simulink model "bicycle"  (R2025b)
settings: Solver=VariableStepAuto  StartTime=0.0  StopTime=10.0  RelTol=1e-3
undefined symbols (not defined in the file): vehicle
settings Model: Creator=jaiden  LastModifiedBy=jaiden

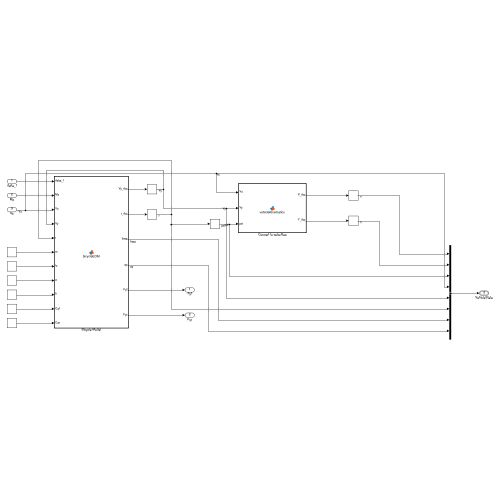
[thumbnail: Simulink's stored preview of the top-level diagram]
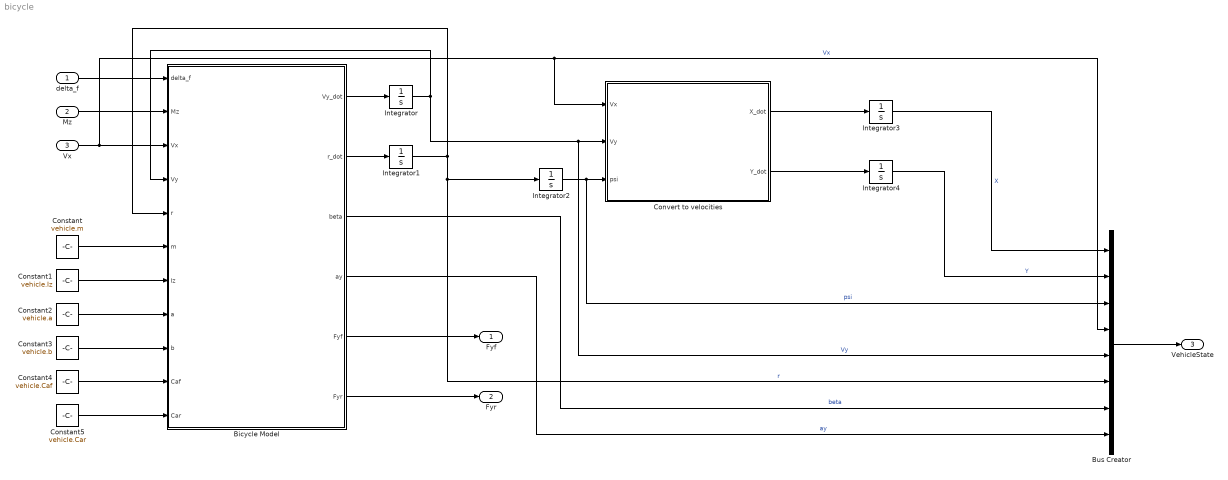
== system bicycle ==
  delta_f : Inport
  Mz : Inport  Port=2
  Vx : Inport  Port=3
  Bicycle Model : MATLAB Function  TreatAsAtomicUnit=on
  Bus Creator : BusCreator  Inputs=8  OutDataTypeStr=Bus: VehicleStateBus
  Constant : Constant  Value=vehicle.m  VectorParams1D=off
  Constant1 : Constant  Value=vehicle.Iz
  Constant2 : Constant  Value=vehicle.a
  Constant3 : Constant  Value=vehicle.b
  Constant4 : Constant  Value=vehicle.Caf
  Constant5 : Constant  Value=vehicle.Car
  Convert to velocities : MATLAB Function  TreatAsAtomicUnit=on
  Integrator{,1..4} (5 alike) : Integrator
  Fyf : Outport
  Fyr : Outport  Port=2
  VehicleState : Outport  Port=3  OutDataTypeStr=Bus: VehicleStateBus
  wires:
  delta_f/1 -> Bicycle Model/1(delta_f)
  Mz/1 -> Bicycle Model/2(Mz)
  Vx/1 -> Bus Creator/4, Convert to velocities/1(Vx), Bicycle Model/3(Vx)  "Vx"
  Bicycle Model/1(Vy_dot) -> Integrator/1
  Integrator/1 -> Bicycle Model/4(Vy), Bus Creator/5, Convert to velocities/2(Vy)  "Vy"
  Bicycle Model/2(r_dot) -> Integrator1/1
  Integrator1/1 -> Bus Creator/6, Integrator2/1, Bicycle Model/5(r)  "r"
  Constant/1 -> Bicycle Model/6(m)
  Constant1/1 -> Bicycle Model/7(Iz)
  Constant2/1 -> Bicycle Model/8(a)
  Constant3/1 -> Bicycle Model/9(b)
  Constant4/1 -> Bicycle Model/10(Caf)
  Constant5/1 -> Bicycle Model/11(Car)
  Bicycle Model/3(beta) -> Bus Creator/7  "beta"
  Bicycle Model/5(Fyf) -> Fyf/1
  Bicycle Model/6(Fyr) -> Fyr/1
  Integrator2/1 -> Bus Creator/3, Convert to velocities/3(psi)  "psi"
  Convert to velocities/1(X_dot) -> Integrator3/1
  Convert to velocities/2(Y_dot) -> Integrator4/1
  Integrator3/1 -> Bus Creator/1  "X"
  Integrator4/1 -> Bus Creator/2  "Y"
  Bus Creator/1 -> VehicleState/1
  Bicycle Model/4(ay) -> Bus Creator/8  "ay"

== matlab function bicycle/Convert to velocities ==
  data: Vx input; X_dot output; Vy input; psi input; Y_dot output
function [X_dot, Y_dot] = vehicleKinematics(Vx, Vy, psi)

X_dot = Vx*cos(psi) - Vy*sin(psi);
Y_dot = Vx*sin(psi) + Vy*cos(psi);

end

== matlab function bicycle/Bicycle Model ==
  data: delta_f input; Vy_dot output; Mz input; Vx input; Vy input; r input; m input; Iz input; a input; b input; Caf input; Car input; r_dot output; beta output; ay output; Fyf output; Fyr output
function [Vy_dot, r_dot, beta, ay, Fyf, Fyr] = bicycleEOM(delta_f, Mz, Vx, Vy, r, m, Iz, a, b, Caf, Car)

% Tire slip angles
alpha_f = delta_f - (Vy + a*r)/Vx;
alpha_r = -(Vy - b*r)/Vx;

% Linear lateral tire forces
Fyf = Caf*alpha_f;
Fyr = Car*alpha_r;

% Vehicle equations of motion
Vy_dot = (Fyf + Fyr)/m - Vx*r;
r_dot  = (a*Fyf - b*Fyr + Mz)/Iz;

% Derived measurements
beta = atan2(Vy, Vx);
ay = Vy_dot + Vx*r;

end
